simulink model "lvrotor2"  (Simulink 7.1)
settings: Solver=ode45  StartTime=0.0  StopTime=10.0  RelTol=1e-3
undefined symbols (not defined in the file or in its folder): cp_nom, lambda_nom, P_wind_base, Pelec_base, Pnom, speed_nom, wind_base
libraries: DRlib x1
settings Model: Creator=lv  LastModifiedBy=lv

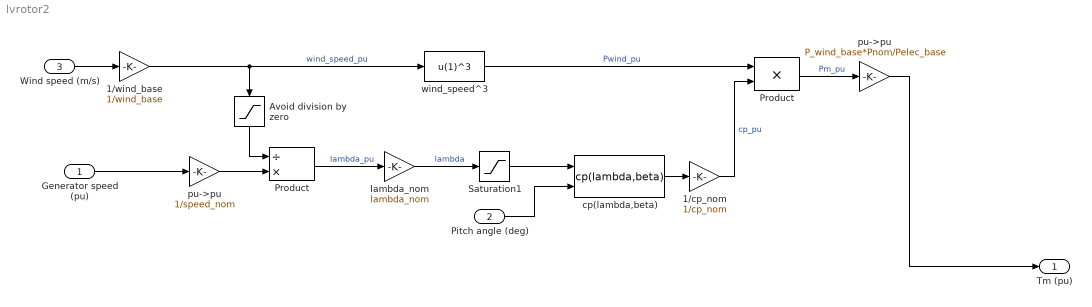
== system lvrotor2 ==
  Generator speed (pu) : Inport  OutDataType=sfix(16)  OutScaling=2^0
  Pitch angle (deg) : Inport  Port=2  OutDataType=sfix(16)  OutScaling=2^0
  Wind speed (m/s) : Inport  Port=3  OutDataType=sfix(16)  OutScaling=2^0
  1/cp_nom : Gain  Gain=1/cp_nom  ParameterDataType=sfix(16)  ParameterScaling=2^0  OutDataType=sfix(16)  OutScaling=2^0  SaturateOnIntegerOverflow=on  OutDataTypeStr=Inherit: Same as input  ParamDataTypeStr=Inherit: Same as input
  1/wind_base : Gain  Gain=1/wind_base  ParameterDataType=sfix(16)  ParameterScaling=2^0  OutDataType=sfix(16)  OutScaling=2^0  SaturateOnIntegerOverflow=on  OutDataTypeStr=Inherit: Same as input  ParamDataTypeStr=Inherit: Same as input
  "Avoid division by zero " : Saturate  Orientation=down  UpperLimit=1e6  LowerLimit=1e-6  OutDataType=sfix(16)  OutScaling=2^0
  Product : Product  Inputs=/*  OutDataType=sfix(16)  OutScaling=2^0  SaturateOnIntegerOverflow=on  OutDataTypeStr=Inherit: Same as first input
  "Product " : Product  OutDataType=sfix(16)  OutScaling=2^0  SaturateOnIntegerOverflow=on  OutDataTypeStr=Inherit: Same as first input
  Saturation1 : Saturate  UpperLimit=inf  LowerLimit=1e-6  OutDataType=sfix(16)  OutScaling=2^0
  cp(lambda,beta) : DRlib/Wind Generation/Wind Turbine/cp(lambda,beta)  SystemSampleTime=-1
  lambda_nom : Gain  Gain=lambda_nom  ParameterDataType=sfix(16)  ParameterScaling=2^0  OutDataType=sfix(16)  OutScaling=2^0  SaturateOnIntegerOverflow=on  OutDataTypeStr=Inherit: Same as input  ParamDataTypeStr=Inherit: Same as input
  pu->pu : Gain  Gain=P_wind_base*Pnom/Pelec_base  ParameterDataType=sfix(16)  ParameterScaling=2^0  OutDataType=sfix(16)  OutScaling=2^0  SaturateOnIntegerOverflow=on  OutDataTypeStr=Inherit: Same as input  ParamDataTypeStr=Inherit: Same as input
  "pu->pu " : Gain  Gain=1/speed_nom  ParameterDataType=sfix(16)  ParameterScaling=2^0  OutDataType=sfix(16)  OutScaling=2^0  SaturateOnIntegerOverflow=on  OutDataTypeStr=Inherit: Same as input  ParamDataTypeStr=Inherit: Same as input
  wind_speed^3 : Fcn  Expr=u(1)^3
  Tm (pu) : Outport  OutDataType=sfix(16)  OutScaling=2^0
  wires:
  Pitch angle (deg)/1 -> cp(lambda,beta)/2
  pu->pu/1 -> Tm (pu)/1
  cp(lambda,beta)/1 -> 1/cp_nom/1
  wind_speed^3/1 -> "Product "/1  "Pwind_pu"
  Wind speed (m/s)/1 -> 1/wind_base/1
  Generator speed (pu)/1 -> "pu->pu "/1
  "Product "/1 -> pu->pu/1  "Pm_pu"
  lambda_nom/1 -> Saturation1/1  "lambda"
  1/cp_nom/1 -> "Product "/2  "cp_pu"
  Saturation1/1 -> cp(lambda,beta)/1
  Product/1 -> lambda_nom/1  "lambda_pu"
  1/wind_base/1 -> wind_speed^3/1, "Avoid division by zero "/1  "wind_speed_pu"
  "Avoid division by zero "/1 -> Product/1
  "pu->pu "/1 -> Product/2
